simulink model "IndustrialMicrogrid"  (R2023a)
settings: Solver=FixedStepDiscrete  StartTime=0.0  StopTime=10  FixedStep=Ts  RelTol=1e-3
PostLoadFcn:
  | IndustrialMicrogridInputData
  | GfmGridFormingConverterInputParameters
model workspace (MAT data in the model file):
  caseNum = 2
undefined symbols (not defined in the file): base, BESS, DiscIntNeverNeededParam, grid, Grid, gridInverter, machine, microgrid, PV, PVInverter, PVTransformer, scrFactorRg, scrFactorXg, transformer, Ts
libraries: ee_lib x112, eeGeneralControl x104, nesl_utility_internal x64, simulink x56, nesl_utility x37, fl_lib x29, slpidlib x13, eeTransforms x11, eeTotalHarmonicDistorsion x8, eeRmsMeasurement x4, eeSinusoidalMeasurement x4, simulink_extras x2
(part 3 of 14)

== system IndustrialMicrogrid/MG1 Primary Substation/Microgrid Controller ==
  note: Microgrid Control Functions
  note: Reference Generation
  note: PLL
  note: PCC Breaker Control
  CntrlRmIN : Inport
  BESS : Inport  Port=2
  "mPCC " : Inport  Port=3
  Active and Reactive Power Reference : Subsystem  mask(Power Reference){PQLowerLimit=microgrid.pqLowerLimit, PQUpperLimit=microgrid.pqUpperLimit}
      mask prompts: PQLowerLimit "PQ Lower Limit"; PQUpperLimit "PQ Upper Limit"
      mask help: Generate active and reactive power reference for BESS
  Black Start : Subsystem  mask(Black Start Control){Controller1BlackStart=microgrid.controller1BlackStart, Controller1BlackStartDelay=microgrid.controller1BlackStartDelay, Controller1BlackStartDelayLevel2=microgrid.controller1BlackStartDelayLevel1, Controller1BlackStartDelayLevel3=microgrid.controller1BlackStartDelayLevel2, Controller1BlackStartVoltageLevel1=microgrid.controller1BlackStartVoltageLevel1, Controller1BlackStartVoltageLevel2=microgrid.controller1BlackStartVoltageLevel2, Controller1BlackStartVoltageLevel3=microgrid.controller1BlackStartVoltageLevel3}
      mask prompts: Controller1BlackStart "Controller 1 Black Start"; Controller1BlackStartDelay "controller 1 Black Start Delay"; Controller1BlackStartDelayLevel2 "Controller 1 Black Start Delay Level 2"; Controller1BlackStartDelayLevel3 "Controller 1 Black Start Delay Level 3"; Controller1BlackStartVoltageLevel1 "Controller 1 Black Start Voltage Level 1"; Controller1BlackStartVoltageLevel2 "Controller 1 Black Start Voltage Level 2"; Controller1BlackStartVoltageLevel3 "Controller 1 Black Start Voltage Level 3"
      mask help: Provide input for black start control
      mask DialogControl ParameterGroupVar Prompt: Parameters
  Breaker Control : Subsystem  mask(Breaker Control){}
      mask help: Control breaker at PCC
  Bus Creator1 : BusCreator  Inputs=3
  Bus Creator2 : BusCreator  Inputs=3
  CntrlRmIN1 : InportShadow
  CntrlRmIN3 : InportShadow
  Frequency Reference : Subsystem  mask(Frequency Reference){GridFrequency=grid.frequency, IslandFrequency=microgrid.islandFrequency}
      mask prompts: GridFrequency "Grid Frequency"; IslandFrequency "Island Frequency"
      mask help: Generate frequency reference for BESS
  PLL : Subsystem  mask(PLL Parameters){KpPLLController1=microgrid.KpPLLController1, KiPLLController1=microgrid.KiPLLController1, GridFrequency=grid.frequency, Ts=Ts}
      mask prompts: KpPLLController1 "PLL Controller 1 Proportional Gain"; KiPLLController1 "PLL Controller 1 Integral Gain"; GridFrequency "Grid Frequency"; Ts "Sampling Time"
      mask help: Provide parameters for PLL
  Planned Island : Subsystem
  Resynchronization : Subsystem
  Voltage Reference : Subsystem  mask(Voltage Reference){IslandVoltage=microgrid.islandVoltage}
      mask prompts: IslandVoltage "Island Voltage"
      mask help: Generate voltage reference for BESS
  PQref : Outport
  Vref : Outport  Port=2
  fref : Outport  Port=3
  MGCtrl : Outport  Port=4
  BreakerControl : Outport  Port=5
  wires:
  Voltage Reference/1(Vref) -> Vref/1
  CntrlRmIN/1 -> Voltage Reference/1(Control Room), Breaker Control/1(Control Room), Frequency Reference/1(Control Room), Active and Reactive Power Reference/1(Control Room)
  [MGController] -> Voltage Reference/2(MGController)
  CntrlRmIN3/1 -> Planned Island/2(Control Room)
  Bus Creator2/1 -> [MGController], MGCtrl/1  "MGController"
  Black Start/1(BlackStartcontroller1) -> Bus Creator2/1  "BlackStart"
  [MGController] -> Active and Reactive Power Reference/2(MGController)
  [MGController] -> Breaker Control/2(MGController)
  Breaker Control/1(BreakerControl) -> BreakerControl/1
  PLL/1(Grid) -> Bus Creator1/1  "Grid"
  [PLL] -> Resynchronization/2(mPCCPLL)
  Active and Reactive Power Reference/1(PQref) -> PQref/1
  Frequency Reference/1(fref) -> fref/1
  "mPCC "/1 -> Bus Creator1/3, PLL/1("mPCC ")  "PCC"
  Resynchronization/1(ResynchMGController) -> Bus Creator2/2
  Planned Island/1(IslandMGController) -> Bus Creator2/3
  Bus Creator1/1 -> [PLL]  "PLL"
  [MGController] -> Frequency Reference/2(MGController)
  PLL/2(Island) -> Bus Creator1/2  "Island"
  CntrlRmIN1/1 -> Resynchronization/1(Control Room), Black Start/1(Control Room)
  BESS/1 -> Resynchronization/3(BESS)
  [PLL] -> Planned Island/1(mPCCPLL)

== system IndustrialMicrogrid/MG1 Primary Substation/PCC Measurements and PCC Breaker ==
  cBreaker : Inport
  Bus Creator : BusCreator  Inputs=2
  Circuit Breaker (Three-Phase) : ee_lib/Switches & Breakers/Circuit Breaker (Three-Phase)  R_closed=0.001 Ohm  G_open=1e-6 1/Ohm  threshold=0.5 V  breaker_behavior=ee.enum.switches.breakerBehavior.zeroCrossingDisable
      settings: InternalSimscapePortConfiguration="{\"Bottom\":[],\"Left\":[{\"id\":\"vT\",\"label\":\"vT\",\"type\":\"input\"},{\"id\":\"N1\",\"label\":\"~1\",\"type\":\"foundation.electrical.three_phase\"}],\"Right\":[{\"id\":\"N2\",\"label\":\"~2\",\"type\":\"foundation.electrical.three_phase\"}],\"Top\":[]}"
  Grid Current Measurement : Subsystem
  Grid Power Measurement : Subsystem
  Simulink-PS Converter : nesl_utility/Simulink-PS Converter  PhysicalDomain=network_engine_domain  SubClassName=ps_input  LeftPortType=input  RightPortType=output  PseudoPeriodic=off  Frequencies=[]  NoiseDistribution=none  NoiseParameters=[]  Unit=1  AffineConversion=off  FilteringAndDerivatives=provide  SimscapeFilterOrder=1  InputFilterTimeConstant=0.001  UdotUserProvided=0
  ~ : PMIOPort  Side=Left
  "~ " : PMIOPort  Port=2  Side=Right
  " mPCC" : Outport
  wires:
  Grid Current Measurement/1("Grid voltage ") -> Bus Creator/1  "Grid voltage"
  Bus Creator/1 -> " mPCC"/1
  Grid Power Measurement/1(mPCC) -> Bus Creator/2  "mPCC"
  cBreaker/1 -> Simulink-PS Converter/1
  connections:
  Grid Current Measurement/RConn1 -- Circuit Breaker (Three-Phase)/LConn2
  Grid Power Measurement/RConn1 -- "~ "/RConn1
  Simulink-PS Converter/RConn1 -- Circuit Breaker (Three-Phase)/LConn1
  Grid Power Measurement/LConn1 -- Circuit Breaker (Three-Phase)/RConn1
  ~/RConn1 -- Grid Current Measurement/LConn1

== system IndustrialMicrogrid/MG1 Primary Substation/Transformer and Disconnectors ==
  Connectors : ee_lib/Passive/RLC Assemblies/RLC (Three-Phase)  component_structure=ee.enum.rlc.structure.R  R=grid.connectorResistance Ohm  L=0.01 H  C=1e-6 F  R_parasitic=1e-6 Ohm  G_parasitic=1e-6 1/Ohm  IL_specify=on  IL_priority=High  IL=[0, 0, 0] A  IL_nominal_specify=off  IL_nominal_unit=A  IL_nominal_value=1  VC_specify=off  VC_priority=High  VC=[0, 0, 0] V  VC_nominal_specify=off  VC_nominal_unit=V  VC_nominal_value=1
      settings: InternalSimscapePortConfiguration="{\"Bottom\":[],\"Left\":[{\"id\":\"N1\",\"label\":\"~1\",\"type\":\"foundation.electrical.three_phase\"}],\"Right\":[{\"id\":\"N2\",\"label\":\"~2\",\"type\":\"foundation.electrical.three_phase\"}],\"Top\":[]}"
  Two-Winding Transformer (Three-Phase)1 : ee_lib/Passive/Transformers/Two-Winding Transformer (Three-Phase)  SRated=grid.transformerRating A*V  FRated=grid.frequency Hz  Winding1Connection=ee.enum.windingconnection.Y  VRated1=grid.transformerPrimaryVoltage V  Winding2Connection=ee.enum.windingconnection.Y  VRated2=grid.transformerSecondaryVoltage V  CoreType=ee.enum.coretype.threelimb  pu_Rw1=grid.primaryResistance  pu_Rw2=grid.primaryReactance  leakage_reactance_option=ee.enum.transformer_leakage.include  pu_Xl1=grid.secondaryResistance  pu_Xl2=grid.secondaryReactance  magnetizing_resistance_option=ee.enum.transformer_magnetizingResistance.include  pu_Rm=500  magnetizing_reactance_option=ee.enum.transformer_magnetizingReactance.include  saturation_option=ee.enum.transformer_saturation.exclude  pu_Xm=500  current_data=[0, .002, 1, 2]  magnetic_flux_data=[0, 1.2, 1.5, 1.51]  pu_X0=0.5  i1_specify=on  i1_priority=None  i1=[0, 0, 0] A  i1_nominal_specify=off  i1_nominal_unit=A  i1_nominal_value=1  i2_specify=on  i2_priority=None  i2=[0, 0, 0] A  i2_nominal_specify=off  i2_nominal_unit=A  i2_nominal_value=1  phi_specify=off  phi_priority=None  phi=[0, 0, 0]  phi_nominal_specify=off  phi_nominal_unit=1  phi_nominal_value=1  power_dissipated_specify=off  power_dissipated_priority=None  power_dissipated=0 W  power_dissipated_nominal_specify=off  power_dissipated_nominal_unit=W  power_dissipated_nominal_value=1
      settings: InternalSimscapePortConfiguration="{\"Bottom\":[],\"Left\":[{\"id\":\"N1\",\"label\":\"~1\",\"type\":\"foundation.electrical.three_phase\"}],\"Right\":[{\"id\":\"N2\",\"label\":\"~2\",\"type\":\"foundation.electrical.three_phase\"}],\"Top\":[]}"
  "~ " : PMIOPort  Side=Right
  ~ : PMIOPort  Port=2  Side=Left
  connections:
  Connectors/LConn1 -- Two-Winding Transformer (Three-Phase)1/RConn1
  Connectors/RConn1 -- "~ "/RConn1
  ~/RConn1 -- Two-Winding Transformer (Three-Phase)1/LConn1

== system IndustrialMicrogrid/MG2 PV Plant/(500KWp PV) ==
  In Bus Element3 : Inport  PortName=Vbus
  Constant : Constant  Value=0  SampleTime=Ts
  Constant1 : Constant  Value=0  SampleTime=Ts
  Constant2 : Constant  Value=1000  VectorParams1D=off  SampleTime=-1
  Current and Voltage Sensor (Three-Phase)3 : ee_lib/Sensors & Transducers/Current and Voltage Sensor (Three-Phase)  vMeasurementType=ee.enum.vmeasurement.lg  outputUnit=ee.enum.unit.pu  SRated=PV.MVABaseNew A*V  VRated=PV.kVBaseNew V  I_specify=off  I_priority=None  I=[0, 0, 0] A  I_nominal_specify=off  I_nominal_unit=A  I_nominal_value=1  V_specify=off  V_priority=None  V=[0, 0, 0] V  V_nominal_specify=off  V_nominal_unit=V  V_nominal_value=1
      settings: InternalSimscapePortConfiguration="{\"Bottom\":[],\"Left\":[{\"id\":\"N1\",\"label\":\"~1\",\"type\":\"foundation.electrical.three_phase\"}],\"Right\":[{\"id\":\"V_output\",\"label\":\"V\",\"type\":\"output\"},{\"id\":\"I_output\",\"label\":\"I\",\"type\":\"output\"},{\"id\":\"N2\",\"label\":\"~2\",\"type\":\"foundation.electrical.three_phase\"}],\"Top\":[]}"
  L Filter2 : ee_lib/Passive/RLC Assemblies/RLC (Three-Phase)  component_structure=ee.enum.rlc.structure.SeriesRL  R=0.1 Ohm  L=PVInverter.l*3 H  C=1e-6 F  R_parasitic=0 Ohm  G_parasitic=0 1/Ohm  IL_specify=off  IL_priority=High  IL=[0, 0, 0] A  IL_nominal_specify=off  IL_nominal_unit=A  IL_nominal_value=1  VC_specify=off  VC_priority=High  VC=[0, 0, 0] V  VC_nominal_specify=off  VC_nominal_unit=V  VC_nominal_value=1
      settings: InternalSimscapePortConfiguration="{\"Bottom\":[],\"Left\":[{\"id\":\"N1\",\"label\":\"~1\",\"type\":\"foundation.electrical.three_phase\"}],\"Right\":[{\"id\":\"N2\",\"label\":\"~2\",\"type\":\"foundation.electrical.three_phase\"}],\"Top\":[]}"
  Low-Pass Filter (Discrete or Continuous) : eeGeneralControl/Low-Pass Filter (Discrete or Continuous)  K=1  T=0.1  B=inf  A=-inf  init_option=Inherited from block input  x0=0  Ts=-1
  Low-Pass Filter (Discrete or Continuous)1 : eeGeneralControl/Low-Pass Filter (Discrete or Continuous)  K=1  T=0.1  B=inf  A=-inf  init_option=Inherited from block input  x0=0  Ts=-1
  Measurement2 : Subsystem
  PS-Simulink Converter : nesl_utility/PS-Simulink Converter  PhysicalDomain=network_engine_domain  SubClassName=ps_output  LeftPortType=input  RightPortType=output  PseudoPeriodic=off  Frequencies=[]  VectorFormat=inherit  Unit=MW  AffineConversion=off
  PS-Simulink Converter2 : nesl_utility/PS-Simulink Converter  PhysicalDomain=network_engine_domain  SubClassName=ps_output  LeftPortType=input  RightPortType=output  PseudoPeriodic=off  Frequencies=[]  VectorFormat=inherit  Unit=MV*A  AffineConversion=off
  PS-Simulink Converter5 : nesl_utility/PS-Simulink Converter  PhysicalDomain=network_engine_domain  SubClassName=ps_output  LeftPortType=input  RightPortType=output  PseudoPeriodic=off  Frequencies=[]  VectorFormat=inherit  Unit=inherit  AffineConversion=off
  PS-Simulink Converter6 : nesl_utility/PS-Simulink Converter  PhysicalDomain=network_engine_domain  SubClassName=ps_output  LeftPortType=input  RightPortType=output  PseudoPeriodic=off  Frequencies=[]  VectorFormat=inherit  Unit=inherit  AffineConversion=off
  PV Inverter A2 : Subsystem
  Power Sensor (Three-Phase) : ee_lib/Sensors & Transducers/Power Sensor (Three-Phase)  load_type=ee.enum.passive.type_balanced.balanced  f0=60 Hz  config=ee.enum.with_neutral.no  rho=1
      settings: InternalSimscapePortConfiguration="{\"Bottom\":[],\"Left\":[{\"id\":\"N1\",\"label\":\"~1\",\"type\":\"foundation.electrical.three_phase\"}],\"Right\":[{\"id\":\"N2\",\"label\":\"~2\",\"type\":\"foundation.electrical.three_phase\"}],\"Top\":[{\"id\":\"Pm\",\"label\":\"P\",\"type\":\"output\"},{\"id\":\"Qm\",\"label\":\"Q\",\"type\":\"output\"}]}"
  Terminator3 : Terminator
  Connection Port : PMIOPort  Side=Left
  Out Bus Element23 : Outport  PortName=mPV  Element=ActivePower
  Out Bus Element1 : Outport  PortName=mPV  Element=RectivePower
  Out Bus Element2 : Outport  PortName=mPV  Element=Voltage
  Out Bus Element3 : Outport  PortName=mPV  Element=Current
  wires:
  Constant2/1 -> PV Inverter A2/1(Insolation)
  Low-Pass Filter (Discrete or Continuous)1/1 -> Out Bus Element23/1
  Low-Pass Filter (Discrete or Continuous)/1 -> Out Bus Element1/1
  PS-Simulink Converter2/1 -> Low-Pass Filter (Discrete or Continuous)/1
  PS-Simulink Converter/1 -> Low-Pass Filter (Discrete or Continuous)1/1
  Constant/1 -> PV Inverter A2/3(LVRT)
  Measurement2/1(ipv1) -> PV Inverter A2/4(ipv1)
  PS-Simulink Converter5/1 -> Out Bus Element3/1, Measurement2/1(u)
  Constant1/1 -> PV Inverter A2/5(Q_ref)
  In Bus Element3/1 -> PV Inverter A2/2(Vbus)
  PS-Simulink Converter6/1 -> Terminator3/1, Out Bus Element2/1
  connections:
  Power Sensor (Three-Phase)/LConn3 -- PS-Simulink Converter2/LConn1
  PS-Simulink Converter/LConn1 -- Power Sensor (Three-Phase)/LConn2
  PV Inverter A2/RConn1 -- Power Sensor (Three-Phase)/LConn1
  L Filter2/LConn1 -- Power Sensor (Three-Phase)/RConn1
  L Filter2/RConn1 -- Current and Voltage Sensor (Three-Phase)3/LConn1
  PS-Simulink Converter6/LConn1 -- Current and Voltage Sensor (Three-Phase)3/RConn1
  PS-Simulink Converter5/LConn1 -- Current and Voltage Sensor (Three-Phase)3/RConn2
  Connection Port/RConn1 -- Current and Voltage Sensor (Three-Phase)3/RConn3

== system IndustrialMicrogrid/MG2 PV Plant/CB4 ==
  Input : Inport
  Circuit Breaker Step off3 : ee_lib/Switches & Breakers/Circuit Breaker (Three-Phase)  R_closed=0.001 Ohm  G_open=1e-4 1/Ohm  threshold=0.5 V  breaker_behavior=ee.enum.switches.breakerBehavior.zeroCrossingEnable
      settings: InternalSimscapePortConfiguration="{\"Bottom\":[],\"Left\":[{\"id\":\"vT\",\"label\":\"vT\",\"type\":\"input\"},{\"id\":\"N1\",\"label\":\"~1\",\"type\":\"foundation.electrical.three_phase\"}],\"Right\":[{\"id\":\"N2\",\"label\":\"~2\",\"type\":\"foundation.electrical.three_phase\"}],\"Top\":[]}"
  Simulink-PS Converter3 : nesl_utility/Simulink-PS Converter  PhysicalDomain=network_engine_domain  SubClassName=ps_input  LeftPortType=input  RightPortType=output  PseudoPeriodic=off  Frequencies=[]  NoiseDistribution=none  NoiseParameters=[]  Unit=1  AffineConversion=off  FilteringAndDerivatives=zero  SimscapeFilterOrder=1  InputFilterTimeConstant=0.001  UdotUserProvided=1
  Conn1 : PMIOPort  Side=Right
  Conn2 : PMIOPort  Port=2  Side=Left
  wires:
  Input/1 -> Simulink-PS Converter3/1
  connections:
  Circuit Breaker Step off3/RConn1 -- Conn1/RConn1
  Circuit Breaker Step off3/LConn1 -- Simulink-PS Converter3/RConn1
  Circuit Breaker Step off3/LConn2 -- Conn2/RConn1

== system IndustrialMicrogrid/MG2 PV Plant/PLL & Measurements2 ==
  V : Inport
  Measurement2 : Subsystem
  PLL : Subsystem
  Out Bus Element : Outport  PortName=Vbus  Element=Vq
  Out Bus Element1 : Outport  PortName=Vbus  Element=Vd
  Out Bus Element2 : Outport  PortName=Vbus  Element=w
  Out Bus Element3 : Outport  PortName=Vbus  Element=Theta
  Out Bus Element4 : Outport  PortName=Vbus  Element=Vmag
  wires:
  V/1 -> Measurement2/1(u)
  PLL/2(freq) -> Out Bus Element2/1
  PLL/5(Vq) -> Out Bus Element/1
  PLL/3(angle) -> Out Bus Element3/1
  PLL/4(Vd) -> Out Bus Element1/1
  Measurement2/1(Vg) -> PLL/1(abc)
  PLL/1(mag) -> Out Bus Element4/1

== system IndustrialMicrogrid/MG2 Power Center/Diesel Generator ==
  AVR and Exciter : Subsystem
  Electrical Reference3 : fl_lib/Electrical/Electrical Elements/Electrical Reference
  "Governor and Prime Mover " : Subsystem  mask(Governor and Prime Mover){pu_speed_reference=machine.speedReference, droop_percentage=machine.droop, pu_load_reference_setpoint=machine.loadReference, T_G=machine.timeConstandGovernor, T_CH=machine.timeConstantPrimeMover, base_torque=machine.baseTorque, pu_torque0=machine.initialTorque}
      mask prompts: pu_speed_reference "Speed reference, (pu)"; droop_percentage "Percentage droop, (%)"; pu_load_reference_setpoint "Load reference setpoint, (pu)"; T_G "Time constant of governor, (s)"; T_CH "Time constant of main inlet volumes and steam chest, (s)"; base_torque "Base torque, (N*m)"; pu_torque0 "Initial torque, (pu)"
      mask help:
      | Implements a synchronous machine governor and prime mover. The prime mover is a non-reheat steam turbine.
      |
      | The input to the block is a per-unit synchronous machine measurement vector.
      |
      | R and C are mechanical rotational ports.
  Machine Inertia : ee_lib/Electromechanical/Mechanical/Machine Inertia  SRated=microgrid.dieselRatedPower V*A  FRated=microgrid.frequency Hz  nPolePairs=1  inertia_option=1  J=0.5754 kg*m^2  H=3.525 s*W/V/A  damper_option=2  D=39.0509 N*m/(rad/s)  pu_D=0.01  initialization_option=2  fMechanical0=60 Hz  fElectrical0=microgrid.frequency Hz
      settings: InternalSimscapePortConfiguration="{\"Bottom\":[],\"Left\":[{\"id\":\"R\",\"label\":\"R\",\"type\":\"foundation.mechanical.rotational.rotational\"}],\"Right\":[],\"Top\":[]}"
  Synchronous Machine Round Rotor : ee_lib/Electromechanical/Synchronous/Synchronous Machine Round Rotor  port_option=ee.enum.threePhasePort.composite  SRated=microgrid.dieselRatedPower A*V  VRated=microgrid.dieselVoltage V  FRated=microgrid.frequency Hz  nPolePairs=1  param_option=ee.enum.sm.parameterization.standard  fieldCircuitParameterization_option=ee.enum.sm.fieldparameterization.current  baseEfd=92.95 V  baseIfd=1300 A  zero_sequence=ee.enum.park.zerosequence.exclude  axes_param=ee.enum.rotorangle.daxis  Ladu=1.66  Laqu=1.61  L0=0.15  Ll=0.05  Ra=0.03  Lfd=0.165  Rfd=0.0006  L1d=0.1713  R1d=0.0284  L1q=0.7252  R1q=0.00619  L2q=0.125  R2q=0.02368  Xl=0.05  Xd=1.72  Xq=0.79  X0=0.06  Xdd=0.13  Xqd=0.17  Xddd=0.09  Xqdd=0.12  d_option=ee.enum.circuit.open  Td0d=0.75 s  Tdd=0.03 s  Td0dd=0.03 s  Tddd=0.008 s  q_option=ee.enum.circuit.open  Tq0d=0.6 s  Tqd=0.03 s  Tq0dd=0.02 s  Tqdd=0.008 s  saturation_option=ee.enum.saturation.exclude  saturation_ifd=[0, .48, .76, 1.38, 1.79]  saturation_Vag=[0, .8, 1.08, 1.31, 1.4]  initialization_option=ee.enum.sm.initialization.steadystate  source_type=ee.enum.sm.load_flow_source_type.Swing  Vmag0=microgrid.dieselVoltage V  Vang0=0 deg  Pt0=0 A*V  Qt0=0 A*V  minimum_pu=0.95  phase_search_range=[-inf, inf] deg  gmin=1e-6 S  connection_option=ee.enum.Connection.wye  num_q_dampers=2  rotor_offset=-pi / 2 rad  pu_psid_specify=off  pu_psid_priority=None  pu_psid=0  pu_psid_nominal_specify=off  pu_psid_nominal_unit=1  pu_psid_nominal_value=1  pu_psiq_specify=off  pu_psiq_priority=None  pu_psiq=0  pu_psiq_nominal_specify=off  pu_psiq_nominal_unit=1  pu_psiq_nominal_value=1  pu_psifd_specify=off  pu_psifd_priority=None  pu_psifd=0  pu_psifd_nominal_specify=off  pu_psifd_nominal_unit=1  pu_psifd_nominal_value=1  pu_psi1d_specify=off  pu_psi1d_priority=None  pu_psi1d=0  pu_psi1d_nominal_specify=off  pu_psi1d_nominal_unit=1  pu_psi1d_nominal_value=1  pu_psi1q_specify=off  pu_psi1q_priority=None  pu_psi1q=0  pu_psi1q_nominal_specify=off  pu_psi1q_nominal_unit=1  pu_psi1q_nominal_value=1  pu_psi2q_specify=off  pu_psi2q_priority=None  pu_psi2q=0  pu_psi2q_nominal_specify=off  pu_psi2q_nominal_unit=1  pu_psi2q_nominal_value=1  angular_position_diff_specify=off  angular_position_diff_priority=None  angular_position_diff=180 deg  angular_position_diff_nominal_specify=off  angular_position_diff_nominal_unit=deg  angular_position_diff_nominal_value=1  Tmeas=298.15 K  alpha=3.93e-3 1/K  stator_thermal_mass=100 J/K  rotor_thermal_mass=200 J/K  temperatureA_specify=off  temperatureA_priority=High  temperatureA=25 degC  temperatureA_nominal_specify=off  temperatureA_nominal_unit=degC  temperatureA_nominal_value=1  temperatureB_specify=off  temperatureB_priority=High  temperatureB=25 degC  temperatureB_nominal_specify=off  temperatureB_nominal_unit=degC  temperatureB_nominal_value=1  temperatureC_specify=off  temperatureC_priority=High  temperatureC=25 degC  temperatureC_nominal_specify=off  temperatureC_nominal_unit=degC  temperatureC_nominal_value=1  temperatureR_specify=off  temperatureR_priority=High  temperatureR=25 degC  temperatureR_nominal_specify=off  temperatureR_nominal_unit=degC  temperatureR_nominal_value=1
      settings: InternalSimscapePortConfiguration="{\"Bottom\":[],\"Left\":[{\"id\":\"fd_p\",\"label\":\"fd+\",\"type\":\"foundation.electrical.electrical\"},{\"id\":\"fd_n\",\"label\":\"fd-\",\"type\":\"foundation.electrical.electrical\"},{\"id\":\"R\",\"label\":\"R\",\"type\":\"foundation.mechanical.rotational.rotational\"},{\"id\":\"C\",\"label\":\"C\",\"type\":\"foundation.mechanical.rotational.rotational\"}],\"Right\":[{\"id\":\"pu_output\",\"label\":\"pu\",\"type\":\"output\"},{\"id\":\"N\",\"label\":\"~\",\"type\":\"foundation.electrical.three_phase\"}],\"Top\":[]}"
  ~ : PMIOPort  Side=Right
  connections:
  ~/RConn1 -- Synchronous Machine Round Rotor/RConn2
  AVR and Exciter/LConn1 -- "Governor and Prime Mover "/LConn1 -- Synchronous Machine Round Rotor/RConn1
  "Governor and Prime Mover "/RConn1 -- Synchronous Machine Round Rotor/LConn3 -- Machine Inertia/LConn1
  Synchronous Machine Round Rotor/LConn1 -- AVR and Exciter/RConn1
  Electrical Reference3/LConn1 -- Synchronous Machine Round Rotor/LConn2 -- AVR and Exciter/RConn2
  Synchronous Machine Round Rotor/LConn4 -- "Governor and Prime Mover "/RConn2

== system IndustrialMicrogrid/MG2 Power Center/Diesel Measurements ==
  Current and Voltage Sensor (Three-Phase)2 : ee_lib/Sensors & Transducers/Current and Voltage Sensor (Three-Phase)  vMeasurementType=ee.enum.vmeasurement.ll  outputUnit=ee.enum.unit.pu  SRated=200e3 A*V  VRated=microgrid.powerCenterVoltage V  I_specify=off  I_priority=None  I=[0, 0, 0] A  I_nominal_specify=off  I_nominal_unit=A  I_nominal_value=1  V_specify=off  V_priority=None  V=[0, 0, 0] V  V_nominal_specify=off  V_nominal_unit=V  V_nominal_value=1
      settings: InternalSimscapePortConfiguration="{\"Bottom\":[],\"Left\":[{\"id\":\"N1\",\"label\":\"~1\",\"type\":\"foundation.electrical.three_phase\"}],\"Right\":[{\"id\":\"V_output\",\"label\":\"V\",\"type\":\"output\"},{\"id\":\"I_output\",\"label\":\"I\",\"type\":\"output\"},{\"id\":\"N2\",\"label\":\"~2\",\"type\":\"foundation.electrical.three_phase\"}],\"Top\":[]}"
  Low-Pass Filter (Discrete or Continuous)1 : eeGeneralControl/Low-Pass Filter (Discrete or Continuous)  K=1  T=0.02  B=inf  A=-inf  init_option=Inherited from block input  x0=0  Ts=Ts
  Low-Pass Filter (Discrete or Continuous)2 : eeGeneralControl/Low-Pass Filter (Discrete or Continuous)  K=1  T=0.02  B=inf  A=-inf  init_option=Inherited from block input  x0=0  Ts=Ts
  PS-Simulink Converter1 : nesl_utility_internal/PS-Simulink Converter  PhysicalDomain=network_engine_domain  SubClassName=ps_output  LeftPortType=input  RightPortType=output  PseudoPeriodic=off  Frequencies=[]  VectorFormat=1-D array  Unit=inherit  AffineConversion=off
  PS-Simulink Converter12 : nesl_utility_internal/PS-Simulink Converter  PhysicalDomain=network_engine_domain  SubClassName=ps_output  LeftPortType=input  RightPortType=output  PseudoPeriodic=off  Frequencies=[]  VectorFormat=inherit  Unit=V  AffineConversion=on
  PS-Simulink Converter13 : nesl_utility_internal/PS-Simulink Converter  PhysicalDomain=network_engine_domain  SubClassName=ps_output  LeftPortType=input  RightPortType=output  PseudoPeriodic=off  Frequencies=[]  VectorFormat=1-D array  Unit=A  AffineConversion=off
  PS-Simulink Converter2 : nesl_utility_internal/PS-Simulink Converter  PhysicalDomain=network_engine_domain  SubClassName=ps_output  LeftPortType=input  RightPortType=output  PseudoPeriodic=off  Frequencies=[]  VectorFormat=1-D array  Unit=inherit  AffineConversion=off
  PS-Simulink Converter6 : nesl_utility_internal/PS-Simulink Converter  PhysicalDomain=network_engine_domain  SubClassName=ps_output  LeftPortType=input  RightPortType=output  PseudoPeriodic=off  Frequencies=[]  VectorFormat=1-D array  Unit=MW  AffineConversion=off
  PS-Simulink Converter7 : nesl_utility_internal/PS-Simulink Converter  PhysicalDomain=network_engine_domain  SubClassName=ps_output  LeftPortType=input  RightPortType=output  PseudoPeriodic=off  Frequencies=[]  VectorFormat=1-D array  Unit=MV*A  AffineConversion=off
  Power Sensor (Three-Phase)1 : ee_lib/Sensors & Transducers/Power Sensor (Three-Phase)  load_type=ee.enum.passive.type_balanced.balanced  f0=60 Hz  config=ee.enum.with_neutral.no  rho=1
      settings: InternalSimscapePortConfiguration="{\"Bottom\":[],\"Left\":[{\"id\":\"N1\",\"label\":\"~1\",\"type\":\"foundation.electrical.three_phase\"}],\"Right\":[{\"id\":\"N2\",\"label\":\"~2\",\"type\":\"foundation.electrical.three_phase\"}],\"Top\":[{\"id\":\"Pm\",\"label\":\"P\",\"type\":\"output\"},{\"id\":\"Qm\",\"label\":\"Q\",\"type\":\"output\"}]}"
  a2 : PMIOPort  Side=Left
  Conn2 : PMIOPort  Port=2  Side=Right
  Out Bus Element : Outport  PortName=mdiesel  Element=active power
  Out Bus Element1 : Outport  PortName=mdiesel  Element=reactive power
  Out Bus Element2 : Outport  PortName=mdiesel  Element=voltage
  Out Bus Element3 : Outport  PortName=mdiesel  Element=current
  Out Bus Element4 : Outport  PortName=mdiesel  Element=voltageRMS
  Out Bus Element5 : Outport  PortName=mdiesel  Element=currentRMS
  wires:
  PS-Simulink Converter12/1 -> Out Bus Element2/1
  PS-Simulink Converter13/1 -> Out Bus Element3/1
  PS-Simulink Converter7/1 -> Low-Pass Filter (Discrete or Continuous)2/1
  PS-Simulink Converter6/1 -> Low-Pass Filter (Discrete or Continuous)1/1
  PS-Simulink Converter1/1 -> Out Bus Element4/1
  PS-Simulink Converter2/1 -> Out Bus Element5/1
  Low-Pass Filter (Discrete or Continuous)1/1 -> Out Bus Element/1
  Low-Pass Filter (Discrete or Continuous)2/1 -> Out Bus Element1/1
  connections:
  Power Sensor (Three-Phase)1/LConn3 -- PS-Simulink Converter7/LConn1
  Power Sensor (Three-Phase)1/LConn2 -- PS-Simulink Converter6/LConn1
  Current and Voltage Sensor (Three-Phase)2/RConn3 -- Conn2/RConn1
  a2/RConn1 -- Power Sensor (Three-Phase)1/LConn1
  Current and Voltage Sensor (Three-Phase)2/RConn1 -- PS-Simulink Converter1/LConn1 -- PS-Simulink Converter12/LConn1
  Current and Voltage Sensor (Three-Phase)2/RConn2 -- PS-Simulink Converter2/LConn1 -- PS-Simulink Converter13/LConn1
  Power Sensor (Three-Phase)1/RConn1 -- Current and Voltage Sensor (Three-Phase)2/LConn1

== system IndustrialMicrogrid/MG2 Power Center/Transformer and Disconnectors ==
  Connectors : ee_lib/Passive/RLC Assemblies/RLC (Three-Phase)  component_structure=ee.enum.rlc.structure.R  R=grid.connectorResistance Ohm  L=0.01 H  C=1e-6 F  R_parasitic=1e-6 Ohm  G_parasitic=1e-6 1/Ohm  IL_specify=on  IL_priority=High  IL=[0, 0, 0] A  IL_nominal_specify=off  IL_nominal_unit=A  IL_nominal_value=1  VC_specify=off  VC_priority=High  VC=[0, 0, 0] V  VC_nominal_specify=off  VC_nominal_unit=V  VC_nominal_value=1
      settings: InternalSimscapePortConfiguration="{\"Bottom\":[],\"Left\":[{\"id\":\"N1\",\"label\":\"~1\",\"type\":\"foundation.electrical.three_phase\"}],\"Right\":[{\"id\":\"N2\",\"label\":\"~2\",\"type\":\"foundation.electrical.three_phase\"}],\"Top\":[]}"
  Electrical Reference5 : fl_lib/Electrical/Electrical Elements/Electrical Reference
  Switchable 10 kW 4160 Vrms 60 Hz1 : ee_lib/Passive/RLC Assemblies/Wye-Connected Load  parameterization=ee.enum.rlc.parameterization.ratedpower  component_structure=ee.enum.rlc.structure.C  component_structure_PQ=ee.enum.rlc.structure.R  R=1 Ohm  L=0.001 H  C=1e-6 F  VRated=microgrid.voltage V  FRated=grid.frequency Hz  P=20000 W  Qpos=0 A*V  Qneg=-30000 A*V  R_parasitic=1e-6 Ohm  G_parasitic=1e-6 1/Ohm  R_parasitic_PQ=1e-6 Ohm  G_parasitic_PQ=1e-6 1/Ohm  Vmag0=microgrid.voltage V  Vang0=0 deg  Freq0=microgrid.frequency Hz  IL_specify=on  IL_priority=High  IL=[ 0 0 0 ] A  IL_nominal_specify=off  IL_nominal_unit=A  IL_nominal_value=1  VC_specify=on  VC_priority=High  VC=[ 0 0 0 ] V  VC_nominal_specify=off  VC_nominal_unit=V  VC_nominal_value=1
  Two-Winding Transformer (Three-Phase)1 : ee_lib/Passive/Transformers/Two-Winding Transformer (Three-Phase)  SRated=microgrid.dieselTransformerRating A*V  FRated=microgrid.frequency Hz  Winding1Connection=ee.enum.windingconnection.Y  VRated1=microgrid.dieselTransformerPrimaryVoltage V  Winding2Connection=ee.enum.windingconnection.Y  VRated2=microgrid.dieselTransformerSecondaryVoltage V  CoreType=ee.enum.coretype.threelimb  pu_Rw1=microgrid.dieselPrimaryResistance  pu_Rw2=microgrid.dieselPrimaryReactance  leakage_reactance_option=ee.enum.transformer_leakage.include  pu_Xl1=microgrid.dieselSecondaryResistance  pu_Xl2=microgrid.dieselSecondaryReactance  magnetizing_resistance_option=ee.enum.transformer_magnetizingResistance.include  pu_Rm=500  magnetizing_reactance_option=ee.enum.transformer_magnetizingReactance.include  saturation_option=ee.enum.transformer_saturation.exclude  pu_Xm=500  current_data=[0, .002, 1, 2]  magnetic_flux_data=[0, 1.2, 1.5, 1.51]  pu_X0=0.5  i1_specify=on  i1_priority=None  i1=[0, 0, 0] A  i1_nominal_specify=off  i1_nominal_unit=A  i1_nominal_value=1  i2_specify=on  i2_priority=None  i2=[0, 0, 0] A  i2_nominal_specify=off  i2_nominal_unit=A  i2_nominal_value=1  phi_specify=off  phi_priority=None  phi=[0, 0, 0]  phi_nominal_specify=off  phi_nominal_unit=1  phi_nominal_value=1  power_dissipated_specify=off  power_dissipated_priority=None  power_dissipated=0 W  power_dissipated_nominal_specify=off  power_dissipated_nominal_unit=W  power_dissipated_nominal_value=1
      settings: InternalSimscapePortConfiguration="{\"Bottom\":[],\"Left\":[{\"id\":\"N1\",\"label\":\"~1\",\"type\":\"foundation.electrical.three_phase\"}],\"Right\":[{\"id\":\"N2\",\"label\":\"~2\",\"type\":\"foundation.electrical.three_phase\"}],\"Top\":[]}"
  ~ : PMIOPort  Side=Left
  "~ " : PMIOPort  Port=2  Side=Right
  connections:
  Two-Winding Transformer (Three-Phase)1/RConn1 -- Connectors/LConn1
  Connectors/RConn1 -- Switchable 10 kW 4160 Vrms 60 Hz1/LConn1 -- "~ "/RConn1
  Two-Winding Transformer (Three-Phase)1/LConn1 -- ~/RConn1
  Switchable 10 kW 4160 Vrms 60 Hz1/RConn1 -- Electrical Reference5/LConn1

== system IndustrialMicrogrid/MG2 Primary Substation/BESS and Controller 2 ==
  CntrlRmIN : Inport
  PQref : Inport  Port=2
  Vref : Inport  Port=3
  f0 : Inport  Port=4
  BESS : Subsystem
      settings: PortSchema="{\"entries\":[{\"content\":{\"sides\":[{\"content\":{\"connectorIds\":[\"LConn1\"]},\"type\":\"ConnectorPlacement.EquallySpacedRectSide\",\"uuid\":\"2696dcad-9c9f-4771-9a46-e4805fbfd4e9\"},{\"content\":{\"connectorIds\":[\"In1\",\"In2\",\"In3\",\"In4\"],\"side\":\"RIGHT\"},\"type\":\"ConnectorPlacement.EquallySpacedRectSide\",\"uuid\":\"645d6df5-6573-4261-af42-019db177e35c\"},{\"content\":{\"side\":\"TOP\"},\"type\":\"ConnectorPlacement.EquallySpacedRectSide\",\"uuid\":\"6dbeb1fb-6f20-4035-89b5-3497a08373ed\"}]},\"type\":\"ConnectorPlacement.EquallySpacedConnector\",\"uuid\":\"8e6ce7c3-5a23-40aa-ad05-ea5cef07dce4\"}],\"packageUris\":[\"http://schema.mathworks.com/mf0/Connector/R2020b\"],\"version\":\"1.0\"}"
  "BESS Converter Measurement " : Subsystem
  BESS output filter and transformer1 : Subsystem
  Circuit Breaker (Three-Phase) : ee_lib/Switches & Breakers/Circuit Breaker (Three-Phase)  R_closed=0.001 Ohm  G_open=1e-6 1/Ohm  threshold=0.5 V  breaker_behavior=ee.enum.switches.breakerBehavior.zeroCrossingEnable
      settings: InternalSimscapePortConfiguration="{\"Bottom\":[],\"Left\":[{\"id\":\"vT\",\"label\":\"vT\",\"type\":\"input\"},{\"id\":\"N1\",\"label\":\"~1\",\"type\":\"foundation.electrical.three_phase\"}],\"Right\":[{\"id\":\"N2\",\"label\":\"~2\",\"type\":\"foundation.electrical.three_phase\"}],\"Top\":[]}"
  Constant : Constant  Value=0
  Simulink-PS Converter : nesl_utility/Simulink-PS Converter  PhysicalDomain=network_engine_domain  SubClassName=ps_input  LeftPortType=input  RightPortType=output  PseudoPeriodic=off  Frequencies=[]  NoiseDistribution=none  NoiseParameters=[]  Unit=1  AffineConversion=off  FilteringAndDerivatives=provide  SimscapeFilterOrder=1  InputFilterTimeConstant=0.001  UdotUserProvided=0
  ~ : PMIOPort  Side=Left
  mBESS : Outport
  wires:
  PQref/1 -> BESS/2(PQref)
  "BESS Converter Measurement "/1(mBESS2) -> mBESS/1
  Vref/1 -> BESS/3(Vref)
  f0/1 -> BESS/4(f0)
  Constant/1 -> Simulink-PS Converter/1
  CntrlRmIN/1 -> BESS/1(CntrlRmIN1)
  connections:
  BESS output filter and transformer1/RConn1 -- "BESS Converter Measurement "/LConn1
  "BESS Converter Measurement "/RConn1 -- Circuit Breaker (Three-Phase)/LConn2
  Circuit Breaker (Three-Phase)/RConn1 -- ~/RConn1
  Simulink-PS Converter/RConn1 -- Circuit Breaker (Three-Phase)/LConn1
  BESS/LConn1 -- BESS output filter and transformer1/LConn1

== system IndustrialMicrogrid/MG2 Primary Substation/Microgrid Controller 2 ==
  note: PCC Breaker Control
  note: PLL
  note: Reference Generation
  note: Microgrid Control Functions
  CntrlRmIN : Inport
  BESS 2 : Inport  Port=2
  "mPCC2 " : Inport  Port=3
  Active and Reactive Power Reference : Subsystem  mask(Power Reference){PQLowerLimit=microgrid.pqLowerLimit, PQUpperLimit=microgrid.pqUpperLimit}
      mask prompts: PQLowerLimit "PQ Lower Limit"; PQUpperLimit "PQ Upper Limit"
      mask help: Generate active and reactive power reference for BESS. Provide upper and lower limit for power references.
  Black Start : Subsystem  mask(Black Start Control){Controller2BlackStart=microgrid.controller2BlackStart, Controller2BlackStartDelay=microgrid.controller2BlackStartDelay, Controller2BlackStartDelayLevel2=microgrid.controller2BlackStartDelayLevel1, Controller2BlackStartDelayLevel3=microgrid.controller2BlackStartDelayLevel2, Controller2BlackStartVoltageLevel1=microgrid.controller2BlackStartVoltageLevel1, Controller2BlackStartVoltageLevel2=microgrid.controller2BlackStartVoltageLevel2, Controller2BlackStartVoltageLevel3=microgrid.controller2BlackStartVoltageLevel3}
      mask prompts: Controller2BlackStart "Controller 2 Black Start"; Controller2BlackStartDelay "Controller 2 Black Start Delay"; Controller2BlackStartDelayLevel2 "Controller 2 Black Start Delay Level 2"; Controller2BlackStartDelayLevel3 "Controller 2 Black Start Delay Level 3"; Controller2BlackStartVoltageLevel1 "Controller 2 Black Start Voltage Level 1"; Controller2BlackStartVoltageLevel2 "Controller 2 Black Start Voltage Level 2"; Controller2BlackStartVoltageLevel3 "Controller 2 Black Start Voltage Level 3"
      mask help: Provide input parameters fro black start control
  "Breaker Control " : Subsystem  mask(Breaker Control){}
      mask help: Control of PCC breaker
  Bus Creator1 : BusCreator  Inputs=3
  Bus Creator2 : BusCreator  Inputs=3
  CntrlRmIN1 : InportShadow
  Frequency Reference : Subsystem  mask(Frequency Reference){GridFrequency=grid.frequency, IslandFrequency=microgrid.islandFrequency}
      mask prompts: GridFrequency "Grid Frequency"; IslandFrequency "Island Frequency"
      mask help: Generate frequency reference for BESS
  "PLL " : Subsystem  mask(Frequency Reference){KpPLLController2=microgrid.KpPLLController2, KIPLLController2=microgrid.KiPLLController2, GridFrequency=grid.frequency, Ts=Ts}
      mask prompts: KpPLLController2 "PLL Controller 2 Proportional Gain"; KIPLLController2 "PLL Controller 2 Intregal Gain"; GridFrequency "Grid Frequency"; Ts "Samplign Time"
      mask help: Generate frequency reference
  Planned Island : Subsystem
  Resynchronization : Subsystem
  Voltage Reference : Subsystem  mask(Voltage Reference){IslandVoltage=microgrid.islandVoltage}
      mask prompts: IslandVoltage "Island Voltage"
      mask help: Generate voltage reference for BESS
  PQref : Outport
  Vref : Outport  Port=2
  fref : Outport  Port=3
  MGCtrl : Outport  Port=4
  BrkCtrl : Outport  Port=5
  wires:
  Bus Creator2/1 -> [MGController], MGCtrl/1  "MGController2"
  Resynchronization/1(ResynchMGController2) -> Bus Creator2/2
  Planned Island/1(IslandMGController2) -> Bus Creator2/3
  "PLL "/2(Island2) -> Bus Creator1/2  "Island2"
  "PLL "/1(Grid2) -> Bus Creator1/1  "Grid2"
  BESS 2/1 -> Resynchronization/3(BESS)
  "mPCC2 "/1 -> Bus Creator1/3, "PLL "/1("mPCC2 ")  "PCC2"
  Voltage Reference/1(Vref) -> Vref/1
  CntrlRmIN1/1 -> Black Start/1(Control Room), Planned Island/1(Control Room), Resynchronization/1(Control Room)
  Black Start/1(BlackStartcontroller2) -> Bus Creator2/1  "BlackStart"
  [MGController] -> Voltage Reference/2(MGController)
  Bus Creator1/1 -> [PLL]  "PLL2"
  [PLL] -> Resynchronization/2(mPCCPLL)
  [PLL] -> Planned Island/2(mPCCPLL 2)
  [MGController] -> "Breaker Control "/2(MGController)
  "Breaker Control "/1(Breaker) -> BrkCtrl/1
  CntrlRmIN/1 -> Voltage Reference/1(Control Room), Frequency Reference/1(Control Room), "Breaker Control "/1(Control Room), Active and Reactive Power Reference/1(Control Room)
  [MGController] -> Active and Reactive Power Reference/2(MGController)
  Active and Reactive Power Reference/1(PQref) -> PQref/1
  Frequency Reference/1(fref) -> fref/1
  [MGController] -> Frequency Reference/2(MGController)

== system IndustrialMicrogrid/MG2 Primary Substation/PCC Measurements and PCC Breaker ==
  cBreaker : Inport
  Bus Creator : BusCreator  Inputs=2
  Circuit Breaker (Three-Phase) : ee_lib/Switches & Breakers/Circuit Breaker (Three-Phase)  R_closed=0.001 Ohm  G_open=1e-6 1/Ohm  threshold=0.5 V  breaker_behavior=ee.enum.switches.breakerBehavior.zeroCrossingDisable
      settings: InternalSimscapePortConfiguration="{\"Bottom\":[],\"Left\":[{\"id\":\"vT\",\"label\":\"vT\",\"type\":\"input\"},{\"id\":\"N1\",\"label\":\"~1\",\"type\":\"foundation.electrical.three_phase\"}],\"Right\":[{\"id\":\"N2\",\"label\":\"~2\",\"type\":\"foundation.electrical.three_phase\"}],\"Top\":[]}"
  Grid Current Measurement : Subsystem
  Grid Power Measurement : Subsystem
  Simulink-PS Converter : nesl_utility/Simulink-PS Converter  PhysicalDomain=network_engine_domain  SubClassName=ps_input  LeftPortType=input  RightPortType=output  PseudoPeriodic=off  Frequencies=[]  NoiseDistribution=none  NoiseParameters=[]  Unit=1  AffineConversion=off  FilteringAndDerivatives=provide  SimscapeFilterOrder=1  InputFilterTimeConstant=0.001  UdotUserProvided=0
  ~ : PMIOPort  Side=Left
  "~ " : PMIOPort  Port=2  Side=Right
  " mPCC2" : Outport
  wires:
  Grid Power Measurement/1(mPCC2) -> Bus Creator/2  "mPCC2"
  Bus Creator/1 -> " mPCC2"/1
  Grid Current Measurement/1("Grid voltage 2 ") -> Bus Creator/1  "Gridvoltage"
  cBreaker/1 -> Simulink-PS Converter/1
  connections:
  ~/RConn1 -- Grid Current Measurement/LConn1
  Grid Power Measurement/LConn1 -- Circuit Breaker (Three-Phase)/RConn1
  Grid Power Measurement/RConn1 -- "~ "/RConn1
  Grid Current Measurement/RConn1 -- Circuit Breaker (Three-Phase)/LConn2
  Simulink-PS Converter/RConn1 -- Circuit Breaker (Three-Phase)/LConn1

== system IndustrialMicrogrid/MG2 Primary Substation/Transformer and Disconnectors ==
  Connectors : ee_lib/Passive/RLC Assemblies/RLC (Three-Phase)  component_structure=ee.enum.rlc.structure.R  R=grid.connectorResistance*100 Ohm  L=0.01 H  C=1e-6 F  R_parasitic=1e-6 Ohm  G_parasitic=1e-6 1/Ohm  IL_specify=on  IL_priority=High  IL=[0, 0, 0] A  IL_nominal_specify=off  IL_nominal_unit=A  IL_nominal_value=1  VC_specify=off  VC_priority=High  VC=[0, 0, 0] V  VC_nominal_specify=off  VC_nominal_unit=V  VC_nominal_value=1
      settings: InternalSimscapePortConfiguration="{\"Bottom\":[],\"Left\":[{\"id\":\"N1\",\"label\":\"~1\",\"type\":\"foundation.electrical.three_phase\"}],\"Right\":[{\"id\":\"N2\",\"label\":\"~2\",\"type\":\"foundation.electrical.three_phase\"}],\"Top\":[]}"
  Two-Winding Transformer (Three-Phase)1 : ee_lib/Passive/Transformers/Two-Winding Transformer (Three-Phase)  SRated=grid.transformerRating A*V  FRated=grid.frequency Hz  Winding1Connection=ee.enum.windingconnection.Y  VRated1=grid.transformerPrimaryVoltage V  Winding2Connection=ee.enum.windingconnection.Y  VRated2=grid.transformerSecondaryVoltage V  CoreType=ee.enum.coretype.threelimb  pu_Rw1=grid.primaryResistance  pu_Rw2=grid.primaryReactance  leakage_reactance_option=ee.enum.transformer_leakage.include  pu_Xl1=grid.secondaryResistance  pu_Xl2=grid.secondaryReactance  magnetizing_resistance_option=ee.enum.transformer_magnetizingResistance.include  pu_Rm=500  magnetizing_reactance_option=ee.enum.transformer_magnetizingReactance.include  saturation_option=ee.enum.transformer_saturation.exclude  pu_Xm=500  current_data=[0, .002, 1, 2]  magnetic_flux_data=[0, 1.2, 1.5, 1.51]  pu_X0=0.5  i1_specify=on  i1_priority=None  i1=[0, 0, 0] A  i1_nominal_specify=off  i1_nominal_unit=A  i1_nominal_value=1  i2_specify=on  i2_priority=None  i2=[0, 0, 0] A  i2_nominal_specify=off  i2_nominal_unit=A  i2_nominal_value=1  phi_specify=off  phi_priority=None  phi=[0, 0, 0]  phi_nominal_specify=off  phi_nominal_unit=1  phi_nominal_value=1  power_dissipated_specify=off  power_dissipated_priority=None  power_dissipated=0 W  power_dissipated_nominal_specify=off  power_dissipated_nominal_unit=W  power_dissipated_nominal_value=1
      settings: InternalSimscapePortConfiguration="{\"Bottom\":[],\"Left\":[{\"id\":\"N1\",\"label\":\"~1\",\"type\":\"foundation.electrical.three_phase\"}],\"Right\":[{\"id\":\"N2\",\"label\":\"~2\",\"type\":\"foundation.electrical.three_phase\"}],\"Top\":[]}"
  "~ " : PMIOPort  Side=Right
  ~ : PMIOPort  Port=2  Side=Left
  connections:
  ~/RConn1 -- Two-Winding Transformer (Three-Phase)1/LConn1
  Connectors/RConn1 -- "~ "/RConn1
  Connectors/LConn1 -- Two-Winding Transformer (Three-Phase)1/RConn1

== system IndustrialMicrogrid/MG2 Processing, Lighting and Auxiliary Loads/Load Measurements1 ==
  Current and Voltage Sensor (Three-Phase)2 : ee_lib/Sensors & Transducers/Current and Voltage Sensor (Three-Phase)  vMeasurementType=ee.enum.vmeasurement.ll  outputUnit=ee.enum.unit.pu  SRated=1e6 A*V  VRated=microgrid.powerCenterVoltage V  I_specify=off  I_priority=None  I=[0, 0, 0] A  I_nominal_specify=off  I_nominal_unit=A  I_nominal_value=1  V_specify=off  V_priority=None  V=[0, 0, 0] V  V_nominal_specify=off  V_nominal_unit=V  V_nominal_value=1
      settings: InternalSimscapePortConfiguration="{\"Bottom\":[],\"Left\":[{\"id\":\"N1\",\"label\":\"~1\",\"type\":\"foundation.electrical.three_phase\"}],\"Right\":[{\"id\":\"V_output\",\"label\":\"V\",\"type\":\"output\"},{\"id\":\"I_output\",\"label\":\"I\",\"type\":\"output\"},{\"id\":\"N2\",\"label\":\"~2\",\"type\":\"foundation.electrical.three_phase\"}],\"Top\":[]}"
  Gain : Gain  Gain=sqrt(2)
  Gain1 : Gain  Gain=sqrt(2)
  Low-Pass Filter (Discrete or Continuous)1 : eeGeneralControl/Low-Pass Filter (Discrete or Continuous)  K=1  T=0.04  B=inf  A=-inf  init_option=Inherited from block input  x0=0  Ts=Ts
  Low-Pass Filter (Discrete or Continuous)2 : eeGeneralControl/Low-Pass Filter (Discrete or Continuous)  K=1  T=0.04  B=inf  A=-inf  init_option=Inherited from block input  x0=0  Ts=Ts
  PS-Simulink Converter1 : nesl_utility_internal/PS-Simulink Converter  PhysicalDomain=network_engine_domain  SubClassName=ps_output  LeftPortType=input  RightPortType=output  PseudoPeriodic=off  Frequencies=[]  VectorFormat=1-D array  Unit=inherit  AffineConversion=off
  PS-Simulink Converter12 : nesl_utility_internal/PS-Simulink Converter  PhysicalDomain=network_engine_domain  SubClassName=ps_output  LeftPortType=input  RightPortType=output  PseudoPeriodic=off  Frequencies=[]  VectorFormat=1-D array  Unit=V  AffineConversion=off
  PS-Simulink Converter13 : nesl_utility_internal/PS-Simulink Converter  PhysicalDomain=network_engine_domain  SubClassName=ps_output  LeftPortType=input  RightPortType=output  PseudoPeriodic=off  Frequencies=[]  VectorFormat=1-D array  Unit=A  AffineConversion=off
  PS-Simulink Converter2 : nesl_utility_internal/PS-Simulink Converter  PhysicalDomain=network_engine_domain  SubClassName=ps_output  LeftPortType=input  RightPortType=output  PseudoPeriodic=off  Frequencies=[]  VectorFormat=1-D array  Unit=inherit  AffineConversion=off
  PS-Simulink Converter6 : nesl_utility_internal/PS-Simulink Converter  PhysicalDomain=network_engine_domain  SubClassName=ps_output  LeftPortType=input  RightPortType=output  PseudoPeriodic=off  Frequencies=[]  VectorFormat=1-D array  Unit=MW  AffineConversion=off
  PS-Simulink Converter7 : nesl_utility_internal/PS-Simulink Converter  PhysicalDomain=network_engine_domain  SubClassName=ps_output  LeftPortType=input  RightPortType=output  PseudoPeriodic=off  Frequencies=[]  VectorFormat=1-D array  Unit=MV*A  AffineConversion=off
  Power Sensor (Three-Phase)1 : ee_lib/Sensors & Transducers/Power Sensor (Three-Phase)  load_type=ee.enum.passive.type_balanced.balanced  f0=60 Hz  config=ee.enum.with_neutral.no  rho=1
      settings: InternalSimscapePortConfiguration="{\"Bottom\":[],\"Left\":[{\"id\":\"N1\",\"label\":\"~1\",\"type\":\"foundation.electrical.three_phase\"}],\"Right\":[{\"id\":\"N2\",\"label\":\"~2\",\"type\":\"foundation.electrical.three_phase\"}],\"Top\":[{\"id\":\"Pm\",\"label\":\"P\",\"type\":\"output\"},{\"id\":\"Qm\",\"label\":\"Q\",\"type\":\"output\"}]}"
  RMS Measurement : eeRmsMeasurement/RMS Measurement  LabelModeActiveChoice=Total  F=60  SpecifyHarmonics=off  K=[0 1 2]  Ts=Ts
      settings: LibrarySourceBlock=|
      | ee_sl_lib/Measurements/RMS
      | Measurement
  RMS Measurement1 : eeRmsMeasurement/RMS Measurement  LabelModeActiveChoice=Total  F=60  SpecifyHarmonics=off  K=[0 1 2]  Ts=Ts
      settings: LibrarySourceBlock=|
      | ee_sl_lib/Measurements/RMS
      | Measurement
  a2 : PMIOPort  Side=Left
  Conn2 : PMIOPort  Port=2  Side=Right
  Out Bus Element : Outport  PortName=mLoad2  Element=active power
  Out Bus Element1 : Outport  PortName=mLoad2  Element=reactive power
  Out Bus Element2 : Outport  PortName=mLoad2  Element=voltage
  Out Bus Element3 : Outport  PortName=mLoad2  Element=current
  Out Bus Element4 : Outport  PortName=mLoad2  Element=voltageRMS
  Out Bus Element5 : Outport  PortName=mLoad2  Element=currentRMS
  wires:
  Low-Pass Filter (Discrete or Continuous)2/1 -> Out Bus Element1/1
  Low-Pass Filter (Discrete or Continuous)1/1 -> Out Bus Element/1
  PS-Simulink Converter2/1 -> RMS Measurement1/1
  PS-Simulink Converter1/1 -> RMS Measurement/1
  PS-Simulink Converter6/1 -> Low-Pass Filter (Discrete or Continuous)1/1
  PS-Simulink Converter7/1 -> Low-Pass Filter (Discrete or Continuous)2/1
  PS-Simulink Converter13/1 -> Out Bus Element3/1
  PS-Simulink Converter12/1 -> Out Bus Element2/1
  RMS Measurement/1 -> Gain/1
  RMS Measurement1/1 -> Gain1/1
  Gain/1 -> Out Bus Element4/1
  Gain1/1 -> Out Bus Element5/1
  connections:
  Power Sensor (Three-Phase)1/RConn1 -- Current and Voltage Sensor (Three-Phase)2/LConn1
  PS-Simulink Converter13/LConn1 -- PS-Simulink Converter2/LConn1 -- Current and Voltage Sensor (Three-Phase)2/RConn2
  PS-Simulink Converter12/LConn1 -- PS-Simulink Converter1/LConn1 -- Current and Voltage Sensor (Three-Phase)2/RConn1
  a2/RConn1 -- Power Sensor (Three-Phase)1/LConn1
  Current and Voltage Sensor (Three-Phase)2/RConn3 -- Conn2/RConn1
  Power Sensor (Three-Phase)1/LConn2 -- PS-Simulink Converter6/LConn1
  Power Sensor (Three-Phase)1/LConn3 -- PS-Simulink Converter7/LConn1
